simulink model "q3"  (R2020b)
settings: Solver=VariableStepAuto  StartTime=0.0  StopTime=10.0  RelTol=1e-3
PreLoadFcn:
  | I=5;
  | Kf=1;
  | PBmax=1500;
  | Rr=1.25;
  | TB=0.01;
  | ctrl=1;
  | g=32.18;
  | m=50;
  | mu=[0 0.4 0.8 0.97 1 0.98 0.96 0.94 0.92 0.9 0.88 0.855 0.83 0.81 0.79 0.77 0.75 0.73 0.72 0.71 0.7]
  | slip=[0 0.05 0.1 0.15000000000000002 0.2 0.25 0.30000000000000004 0.35000000000000003 0.4 0.45 0.5 0.55 0.6 0.64999999999999991 0.7 0.75 0.8 0.85 0.9 0.95 1]
  | v0=88
settings Model: OrderedModelArguments=off  Creator=Ravi  LastModifiedBy=Ravi

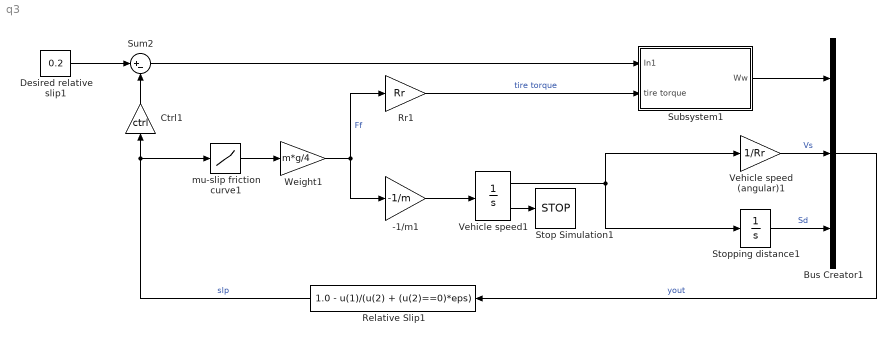
== system q3 ==
  -1/m1 : Gain  Gain=-1/m  SaturateOnIntegerOverflow=on  OutDataTypeStr=Inherit: Same as input  ParamDataTypeStr=Inherit: Same as input
  Bus Creator1 : BusCreator  Inputs=3
  Ctrl1 : Gain  Gain=ctrl  SaturateOnIntegerOverflow=on  OutDataTypeStr=Inherit: Same as input  ParamDataTypeStr=Inherit: Same as input
  Desired relative slip1 : Constant  Value=0.2
  Relative Slip1 : Fcn  Expr=1.0 - u(1)/(u(2) + (u(2)==0)*eps)
  Rr1 : Gain  Gain=Rr  SaturateOnIntegerOverflow=on  OutDataTypeStr=Inherit: Same as input  ParamDataTypeStr=Inherit: Same as input
  Stop Simulation1 : Stop
  Stopping distance1 : Integrator  UpperSaturationLimit=1000  LowerSaturationLimit=0
  Subsystem1 : Subsystem
  Sum2 : Sum  Inputs=|+-  InputSameDT=on  SaturateOnIntegerOverflow=on  OutDataTypeStr=Inherit: Same as first input
  Vehicle speed1 : Integrator  InitialCondition=v0  LimitOutput=on  UpperSaturationLimit=1000  LowerSaturationLimit=0  ShowSaturationPort=on
  Vehicle speed (angular)1 : Gain  Gain=1/Rr  SaturateOnIntegerOverflow=on  OutDataTypeStr=Inherit: Same as input  ParamDataTypeStr=Inherit: Same as input
  Weight1 : Gain  Gain=m*g/4  SaturateOnIntegerOverflow=on  OutDataTypeStr=Inherit: Same as input  ParamDataTypeStr=Inherit: Same as input
  mu-slip friction curve1 : Lookup_n-D  NumberOfTableDimensions=1  BreakpointsForDimension1=slip  Table=mu  SaturateOnIntegerOverflow=on  InputSameDT=on
  wires:
  Subsystem1/1(Ww) -> Bus Creator1/1
  Rr1/1 -> Subsystem1/2(tire torque)  "tire torque"
  Ctrl1/1 -> Sum2/2
  Stopping distance1/1 -> Bus Creator1/3  "Sd"
  Bus Creator1/1 -> Relative Slip1/1  "yout"
  Vehicle speed (angular)1/1 -> Bus Creator1/2  "Vs"
  Vehicle speed1/2 -> Stop Simulation1/1
  Relative Slip1/1 -> Ctrl1/1, mu-slip friction curve1/1  "slp"
  Vehicle speed1/1 -> Stopping distance1/1, Vehicle speed (angular)1/1
  Sum2/1 -> Subsystem1/1(In1)
  mu-slip friction curve1/1 -> Weight1/1
  Weight1/1 -> -1/m1/1, Rr1/1  "Ff"
  Desired relative slip1/1 -> Sum2/1
  -1/m1/1 -> Vehicle speed1/1

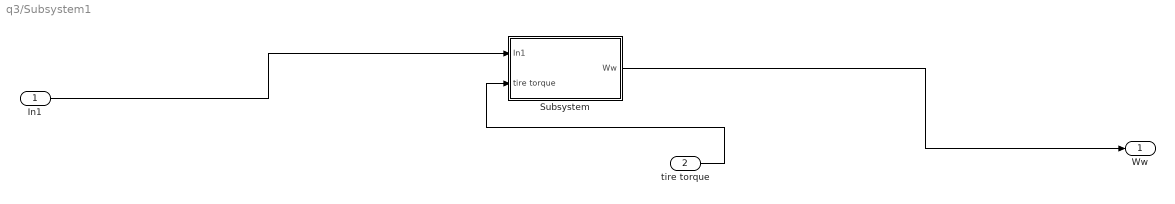
== system q3/Subsystem1 ==
  In1 : Inport
  tire torque : Inport  Port=2
  Subsystem : Subsystem
  Ww : Outport
  wires:
  tire torque/1 -> Subsystem/2(tire torque)
  Subsystem/1(Ww) -> Ww/1
  In1/1 -> Subsystem/1(In1)

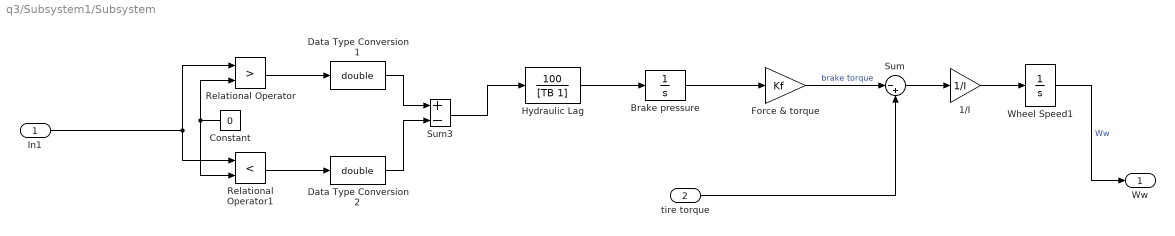
== system q3/Subsystem1/Subsystem ==
  In1 : Inport
  tire torque : Inport  Port=2
  1/I : Gain  Gain=1/I  SaturateOnIntegerOverflow=on  OutDataTypeStr=Inherit: Same as input  ParamDataTypeStr=Inherit: Same as input
  Brake pressure : Integrator  LimitOutput=on  UpperSaturationLimit=PBmax  LowerSaturationLimit=0
  Constant : Constant  Value=0
  Data Type Conversion1 : DataTypeConversion  OutDataTypeStr=double  SaturateOnIntegerOverflow=on  RndMeth=Zero
  Data Type Conversion2 : DataTypeConversion  OutDataTypeStr=double  SaturateOnIntegerOverflow=on  RndMeth=Zero
  Force & torque : Gain  Gain=Kf  SaturateOnIntegerOverflow=on  OutDataTypeStr=Inherit: Same as input  ParamDataTypeStr=Inherit: Same as input
  "Hydraulic Lag " : TransferFcn  Numerator=[100]  Denominator=[TB 1]
  Relational Operator : RelationalOperator  Operator=>  OutDataTypeStr=boolean  RndMeth=Nearest  InputSameDT=on
  Relational Operator1 : RelationalOperator  Operator=<  OutDataTypeStr=boolean  RndMeth=Nearest  InputSameDT=on
  Sum : Sum  Inputs=|-+  InputSameDT=on  SaturateOnIntegerOverflow=on  OutDataTypeStr=Inherit: Same as first input
  Sum3 : Sum  Inputs=+-  InputSameDT=on  SaturateOnIntegerOverflow=on  OutDataTypeStr=Inherit: Same as first input
  Wheel Speed1 : Integrator  InitialCondition=v0/Rr  LimitOutput=on  UpperSaturationLimit=1000  LowerSaturationLimit=0
  Ww : Outport
  wires:
  Sum3/1 -> "Hydraulic Lag "/1
  Relational Operator1/1 -> Data Type Conversion2/1
  In1/1 -> Relational Operator/1, Relational Operator1/1
  Constant/1 -> Relational Operator1/2, Relational Operator/2
  Data Type Conversion2/1 -> Sum3/2
  Force & torque/1 -> Sum/1  "brake torque"
  "Hydraulic Lag "/1 -> Brake pressure/1
  1/I/1 -> Wheel Speed1/1
  Data Type Conversion1/1 -> Sum3/1
  Sum/1 -> 1/I/1
  Relational Operator/1 -> Data Type Conversion1/1
  Brake pressure/1 -> Force & torque/1
  Wheel Speed1/1 -> Ww/1  "Ww"
  tire torque/1 -> Sum/2
